simulink model "gbetest"  (Simulink 7.4)
settings: Solver=ode45  StartTime=0.0  StopTime=10.0  RelTol=1e-3
undefined symbols (not defined in the file or in its folder): BEE2_ctrl
libraries: xps_library x5, xbsIndex_r4 x4
settings Model: Creator=tfiliba  LastModifiedBy=tfiliba

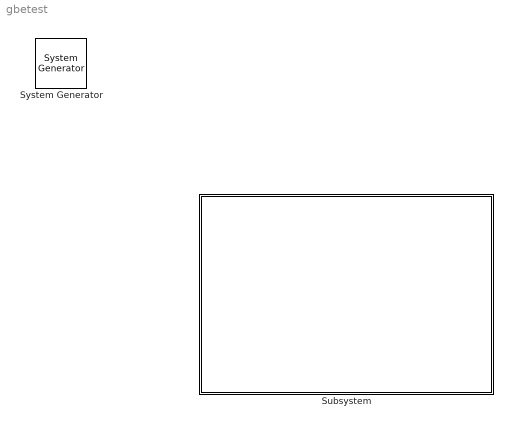
== system gbetest ==
  " System Generator" : xbsIndex_r4/ System Generator  Tag=genX  SystemSampleTime=-1  xilinxfamily=Virtex6  part=xc6vsx315t  speed=-3  package=ff1156  synthesis_tool=XST  clock_wrapper=Clock Enables  directory=./netlist  testbench=off  simulink_period=1  sysclk_period=10  dcm_input_clock_period=10  incr_netlist=off  trim_vbits=Everywhere in SubSystem  dbl_ovrd=According to Block Masks  core_generation=According to Block Masks  run_coregen=off  deprecated_control=off  eval_field=0  block_type=sysgen
      settings: block_version=11.4
  Subsystem : Subsystem
      mask init:
      | cfg.source = str2func('gbetest_init');
      | cfg.toplevel = gcb;
      | cfg.depend = {'gbetest_init'};
      | args = {};
      | xBlock(cfg, args);

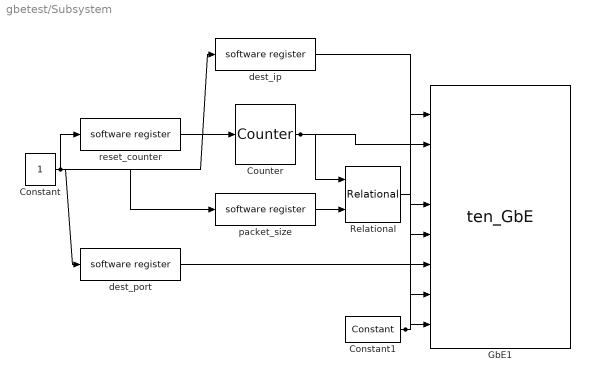
== system gbetest/Subsystem ==
  Constant : Constant  OutDataType=fixdt(1, 16)  OutScaling=2^0
  Constant1 : xbsIndex_r4/Constant  arith_type=Boolean  const=0  n_bits=16  bin_pt=14  explicit_period=off  period=1  equ=P=C  opselect=C  inp2=PCIN>>17  opr=+  inp1=P  carry=CIN  dbl_ovrd=off  block_type=constant
      settings: block_version=11.4
  Counter : xbsIndex_r4/Counter  cnt_type=Free Running  cnt_to=Inf  operation=Up  start_count=0  cnt_by_val=1  arith_type=Unsigned  n_bits=8  bin_pt=0  load_pin=off  rst=on  en=off  explicit_period=on  period=1  dbl_ovrd=off  use_behavioral_HDL=off  implementation=Fabric  block_type=counter
      settings: block_version=11.4
  GbE1 : xps_library/ten_GbE  Tag=xps:tengbe  SystemSampleTime=-1  port=BEE2_ctrl:0  mac_lite=off  open_phy=off  show_param=off  pre_emph=3  swing=800  fab_en=off  fab_mac=0  fab_ip=0  fab_udp=0  fab_gate=0
  Relational : xbsIndex_r4/Relational  mode=a=b  en=off  latency=1  dbl_ovrd=off  block_type=relational
  dest_ip : xps_library/software register  Tag=xps:sw_reg  SystemSampleTime=-1  io_dir=From Processor  arith_type=Unsigned  bitwidth=32  bin_pt=0  sample_period=1  gw_name=gbetest_Subsystem_dest_ip_user_data_out
  dest_port : xps_library/software register  Tag=xps:sw_reg  SystemSampleTime=-1  io_dir=From Processor  arith_type=Unsigned  bitwidth=32  bin_pt=0  sample_period=1  gw_name=gbetest_Subsystem_dest_port_user_data_out
  packet_size : xps_library/software register  Tag=xps:sw_reg  SystemSampleTime=-1  io_dir=From Processor  arith_type=Unsigned  bitwidth=32  bin_pt=0  sample_period=1  gw_name=gbetest_Subsystem_packet_size_user_data_out
  reset_counter : xps_library/software register  Tag=xps:sw_reg  SystemSampleTime=-1  io_dir=From Processor  arith_type=Unsigned  bitwidth=32  bin_pt=0  sample_period=1  gw_name=gbetest_Subsystem_reset_counter_user_data_out
  wires:
  Constant/1 -> packet_size/1, reset_counter/1, dest_port/1, dest_ip/1
  Counter/1 -> GbE1/2, Relational/1
  Constant1/1 -> GbE1/8, GbE1/7, GbE1/1
  Relational/1 -> GbE1/6
  dest_port/1 -> GbE1/5
  dest_ip/1 -> GbE1/4
  packet_size/1 -> Relational/2
  reset_counter/1 -> Counter/1
